simulink model "OutputToStimulatorMultiSite"  (R2016b)
settings: Solver=FixedStepDiscrete  StartTime=0.0  StopTime=inf  FixedStep=sCoreParams.core.stepPeriod  RelTol=1e-3
undefined symbols (not defined in the file): sCoreParams, sCoreParams_stimulator_refractoryPeriodSec, sCoreParams_stimulator_startupTimeSec
libraries: commutil2 x1, xpcparallelportlib x1
Description:
  | This model consists of the simulator configuration and the output to the parallel port.
  | Inputs:
  |   1. isEventDetected: 1 if event was detected 0 if NO event.
  |   2. sendStimPulse: 1 if a stimulus should be sent
  | An example of the usage if this two inputs follows. We could have 2 reason to perform a stimulation (e.g. event detected or sham).
  | In that case input 1 will be 1 only when event is detected while input 2 will be 1 for both stimulations.
  | 
  | Outputs:
  |   1. StimHappening: Indicates that a stimulation pulse was sent through the parallel port to the cerexstim
settings Model: DataTypeOverride=Double  MinMaxOverflowLogging=ForceOff  Creator=rzelmann  LastModifiedBy=rzelmann
settings SolverCC: EnableConcurrentExecution=on  AutoInsertRateTranBlk=on
settings DataIOCC: LimitDataPoints=on  SaveFormat=StructureWithTime  SaveOutput=off  SignalLogging=off  SaveTime=off
settings OptimizationCC: BlockReduction=off  DefaultParameterBehavior=Inlined  OptimizeBlockIOStorage=off  BufferReuse=off  GlobalBufferReuse=off  ExpressionFolding=off  LocalBlockOutputs=off  LifeSpan=inf
settings DebuggingCC: AlgebraicLoopMsg=error  SingleTaskRateTransMsg=error  AllowSymbolicDim=off  SFUnexpectedBacktrackingDiag=warning  SFNoUnconditionalDefaultTransitionDiag=warning  SFExecutionAtInitializationDiag=none
settings HardwareCC: ProdBitPerPointer=32  ProdBitPerSizeT=32  ProdBitPerPtrDiffT=32  ProdLargestAtomicFloat=None  ProdWordSize=32  ProdLongLongMode=on  ProdHWDeviceType=Generic->32-bit x86 compatible
settings ModelReferenceCC: ModelReferenceNumInstancesAllowed=Single  ModelReferencePassRootInputsByReference=off
settings RTWCC: SystemTargetFile=slrt.tlc  TemplateMakefile=slrt_default_tmf  Description=Simulink Real-Time  RTWCompilerOptimization=on
settings ConfigComp: CovMetricSettings=dw  CovHtmlReporting=on  CovSaveCumulativeToWorkspaceVar=on  CovSaveSingleToWorkspaceVar=on  CovExternalEMLEnable=off

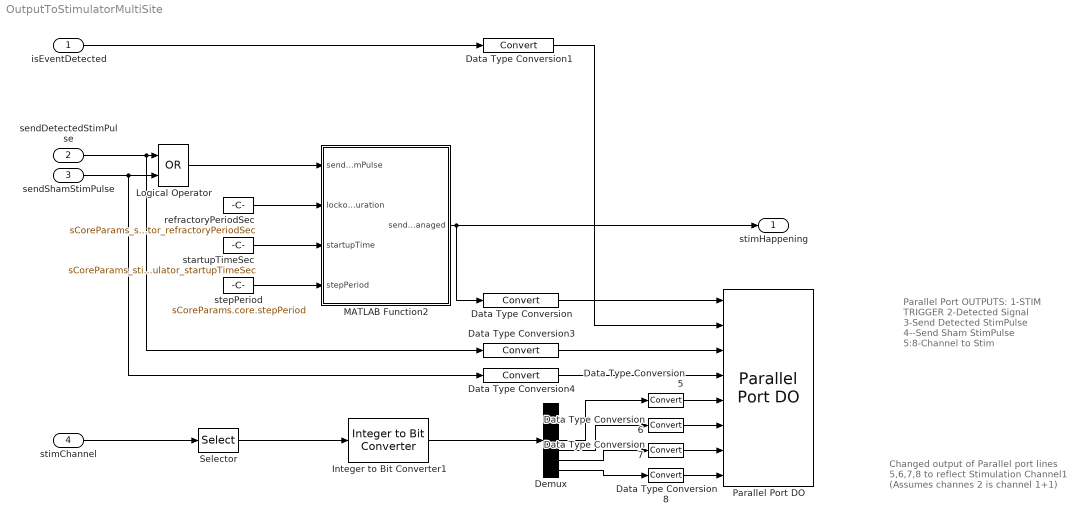
== system OutputToStimulatorMultiSite ==
  note: Parallel Port OUTPUTS:
      | 1-STIM TRIGGER
      | 2-Detected Signal
      | 3-Send Detected StimPulse
      | 4--Send Sham StimPulse
      |
      | 5:8-Channel to Stim
  note: Changed output of Parallel port
      | lines 5,6,7,8
      | to reflect Stimulation Channel1
      | (Assumes channes 2 is channel 1+1)
  isEventDetected : Inport  OutDataTypeStr=boolean  SampleTime=sCoreParams.core.stepPeriod
  sendDetectedStimPulse : Inport  Port=2  OutDataTypeStr=boolean  SampleTime=sCoreParams.core.stepPeriod
  sendShamStimPulse : Inport  Port=3  OutDataTypeStr=boolean  SampleTime=sCoreParams.core.stepPeriod
  stimChannel : Inport  Port=4  OutDataTypeStr=int32  PortDimensions=2  SampleTime=sCoreParams.core.stepPeriod
  Data Type Conversion{,1,3..8} (8 alike) : DataTypeConversion
  Demux : Demux  Outputs=7
  Integer to Bit Converter1 : commutil2/Integer to Bit Converter  nbits=7  signedInputValues=Unsigned  bitOrder=MSB first  outDtype=Inherit via internal rule
  Logical Operator : Logic  Operator=OR  IconShape=distinctive  AllPortsSameDT=off  OutDataTypeStr=boolean
  MATLAB Function2 : MATLAB Function  TreatAsAtomicUnit=on  SystemSampleTime=sCoreParams.core.stepPeriod
  "Parallel Port DO " : xpcparallelportlib/Digital Output/Parallel Port DO   BaseMask=0x378  BaseString=0x378  Format=8 1-bit Channels  Channels=[1:8]  InitialValues=[0]  FinalActions=[0]  FinalValues=[0]  SampleTime=sCoreParams.core.stepPeriod  Mode=1
  Selector : Selector  InputPortWidth=2  IndexOptions=Index vector (dialog)  Indices=[1]  OutputSizes=1
  refractoryPeriodSec : Constant  Value=sCoreParams_stimulator_refractoryPeriodSec
  startupTimeSec : Constant  Value=sCoreParams_stimulator_startupTimeSec
  stepPeriod : Constant  Value=sCoreParams.core.stepPeriod
  stimHappening : Outport  OutDataTypeStr=boolean  SampleTime=sCoreParams.core.stepPeriod
  wires:
  stepPeriod/1 -> MATLAB Function2/4(stepPeriod)
  startupTimeSec/1 -> MATLAB Function2/3(startupTime)
  refractoryPeriodSec/1 -> MATLAB Function2/2(lockoutDuration)
  Data Type Conversion/1 -> "Parallel Port DO "/1
  MATLAB Function2/1(sendStimManaged) -> stimHappening/1, Data Type Conversion/1
  isEventDetected/1 -> Data Type Conversion1/1
  Data Type Conversion1/1 -> "Parallel Port DO "/2
  Data Type Conversion3/1 -> "Parallel Port DO "/3
  stimChannel/1 -> Selector/1
  Demux/4 -> Data Type Conversion5/1
  Demux/5 -> Data Type Conversion6/1
  Demux/6 -> Data Type Conversion7/1
  Demux/7 -> Data Type Conversion8/1
  sendDetectedStimPulse/1 -> Data Type Conversion3/1, Logical Operator/1
  sendShamStimPulse/1 -> Data Type Conversion4/1, Logical Operator/2
  Logical Operator/1 -> MATLAB Function2/1(sendStimPulse)
  Data Type Conversion4/1 -> "Parallel Port DO "/4
  Selector/1 -> Integer to Bit Converter1/1
  Data Type Conversion5/1 -> "Parallel Port DO "/5
  Data Type Conversion6/1 -> "Parallel Port DO "/6
  Data Type Conversion7/1 -> "Parallel Port DO "/7
  Data Type Conversion8/1 -> "Parallel Port DO "/8
  Integer to Bit Converter1/1 -> Demux/1

== matlab function OutputToStimulatorMultiSite/MATLAB Function2 ==
  data: sendStimPulse input; sendStimManaged output; lockoutDuration input; startupTime input; stepPeriod input
function sendStimManaged = ManageStimLockout(sendStimPulse,lockoutDuration,startupTime,stepPeriod)
%#codegen

sendStimManaged = ManageStimLockout_EML(sendStimPulse,lockoutDuration,startupTime,stepPeriod);
%sendStimManaged = double(sendStimManagedB);
